simulink model "Progetto10sml"  (R2016b)
settings: Solver=VariableStepAuto  StartTime=0.0  StopTime=10  RelTol=1e-3
libraries: cstblocks x9
settings Model: Creator=Nicola  LastModifiedBy=Nicola

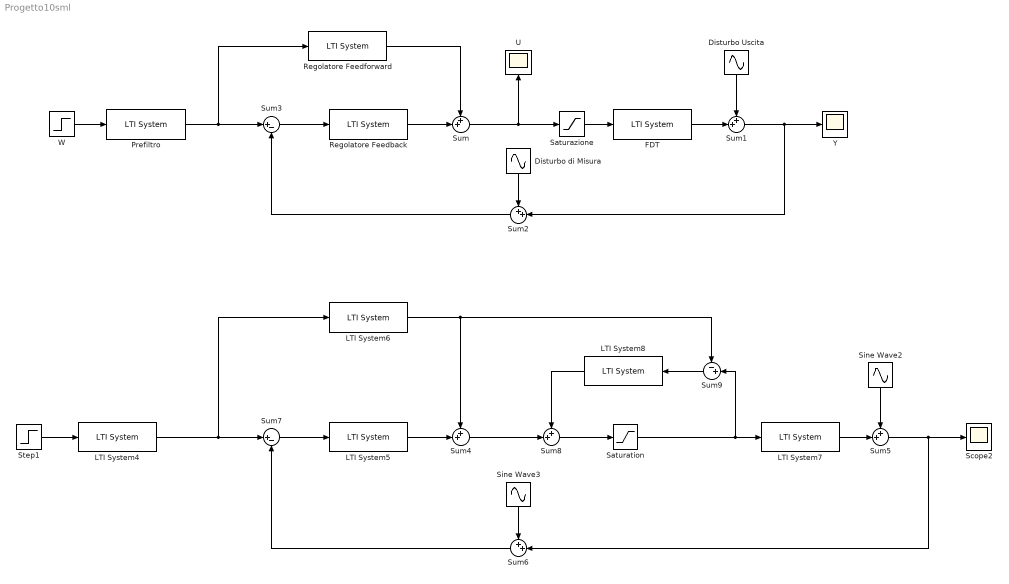
== system Progetto10sml ==
  Disturbo Uscita : Sin  Amplitude=0.3  Frequency=0.08  SampleTime=0
  Disturbo di Misura : Sin  Amplitude=0.02  Frequency=100  SampleTime=0
  FDT : cstblocks/LTI System  sys=G  IC=[]
  LTI System4 : cstblocks/LTI System  sys=Rpf  IC=[]
  LTI System5 : cstblocks/LTI System  sys=aw1  IC=[]
  LTI System6 : cstblocks/LTI System  sys=Rff  IC=[]
  LTI System7 : cstblocks/LTI System  sys=G  IC=[]
  LTI System8 : cstblocks/LTI System  sys=aw2  IC=[]
  Prefiltro : cstblocks/LTI System  sys=Rpf  IC=[]
  Regolatore Feedback : cstblocks/LTI System  sys=Rfb  IC=[]
  Regolatore Feedforward : cstblocks/LTI System  sys=Rff  IC=[]
  Saturation : Saturate  UpperLimit=28.5  LowerLimit=-28.5
  Saturazione : Saturate  UpperLimit=24  LowerLimit=-24
  Scope2 : Scope
  Sine Wave2 : Sin  Amplitude=0.3  Frequency=0.08  SampleTime=0
  Sine Wave3 : Sin  Amplitude=0.02  Frequency=100  SampleTime=0
  Step1 : Step  Time=0  After=2  SampleTime=0
  Sum{,1..2,4..6,8} (7 alike) : Sum  Inputs=++|
  Sum3 : Sum  Inputs=|+-
  Sum7 : Sum  Inputs=|+-
  Sum9 : Sum  Inputs=-+|
  U : Scope
  W : Step  Time=0  After=2  SampleTime=0
  Y : Scope
  wires:
  W/1 -> Prefiltro/1
  Prefiltro/1 -> Sum3/1, Regolatore Feedforward/1
  Regolatore Feedforward/1 -> Sum/1
  Regolatore Feedback/1 -> Sum/2
  Sum/1 -> Saturazione/1, U/1
  Disturbo Uscita/1 -> Sum1/1
  FDT/1 -> Sum1/2
  Sum1/1 -> Sum2/2, Y/1
  Sum2/1 -> Sum3/2
  Sum3/1 -> Regolatore Feedback/1
  Disturbo di Misura/1 -> Sum2/1
  Step1/1 -> LTI System4/1
  LTI System4/1 -> Sum7/1, LTI System6/1
  LTI System6/1 -> Sum9/1, Sum4/1
  LTI System5/1 -> Sum4/2
  Sine Wave2/1 -> Sum5/1
  LTI System7/1 -> Sum5/2
  Sum5/1 -> Sum6/2, Scope2/1
  Sum6/1 -> Sum7/2
  Sum7/1 -> LTI System5/1
  Sine Wave3/1 -> Sum6/1
  Saturation/1 -> Sum9/2, LTI System7/1
  Sum8/1 -> Saturation/1
  Sum4/1 -> Sum8/2
  LTI System8/1 -> Sum8/1
  Sum9/1 -> LTI System8/1
  Saturazione/1 -> FDT/1
